simulink model "smP4"  (R2023a)
settings: Solver=FixedStepAuto  StartTime=0.0  StopTime=10.0  FixedStep=1e-3  RelTol=1e-3
model workspace (MAT data in the model file):
  k = 100
  m = 10
  r = 0.05

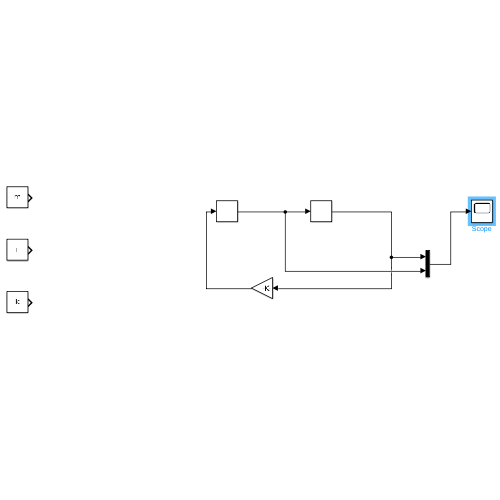
[thumbnail: Simulink's stored preview of the top-level diagram]
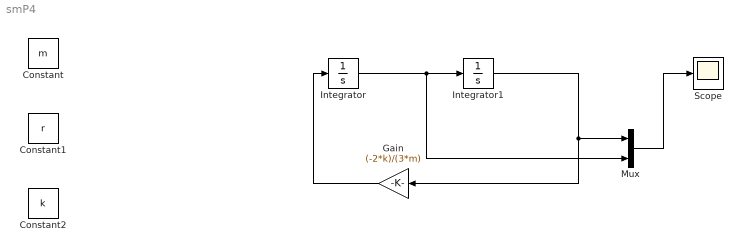
== system smP4 ==
  Constant : Constant  Value=m
  Constant1 : Constant  Value=r
  Constant2 : Constant  Value=k
  Gain : Gain  Gain=(-2*k)/(3*m)
  Integrator : Integrator  InitialCondition=2
  Integrator1 : Integrator
  Mux : Mux  Inputs=2
  Scope : Scope
  wires:
  Integrator/1 -> Mux/2, Integrator1/1
  Integrator1/1 -> Mux/1, Gain/1
  Gain/1 -> Integrator/1
  Mux/1 -> Scope/1
